simulink model "transmitDSSS_singleUser_USRP"  (R2017a)
settings: Solver=VariableStepAuto  StartTime=0.0  StopTime=inf  RelTol=1e-3
InitFcn:
  | Tb = 1/1000;
  | Tc = 1/8000;
  | fs = 64e3;
  | Ts = 1/fs;
libraries: commfilt2 x2, dspsrcs4 x2, commdigbbndpm3 x1, commsdrhw_v2 x1
settings Model: Creator=prust  LastModifiedBy=prust

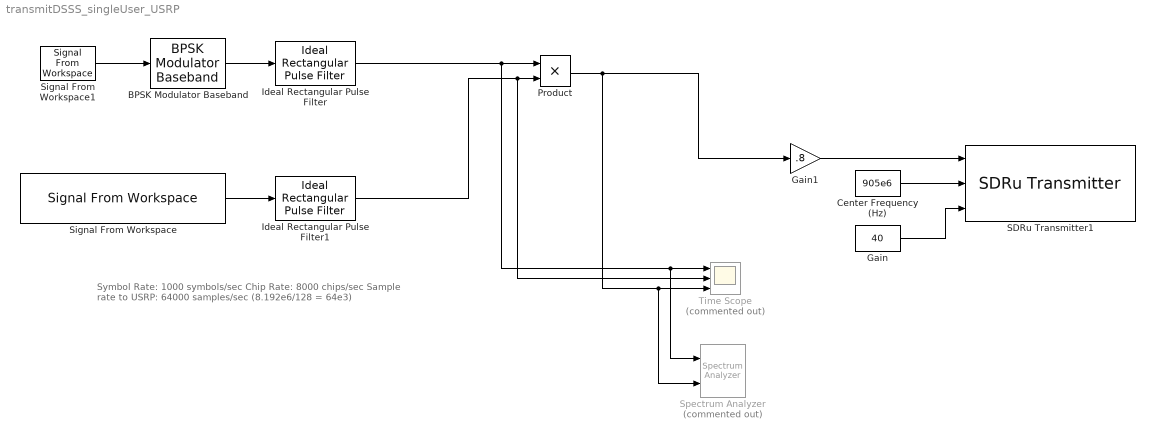
== system transmitDSSS_singleUser_USRP ==
  note: Symbol Rate: 1000 symbols/sec
      | Chip Rate: 8000 chips/sec
      |
      | Sample rate to USRP: 64000 samples/sec
      | (8.192e6/128 = 64e3)
  BPSK Modulator Baseband : commdigbbndpm3/BPSK Modulator Baseband  Ph=0  outDtype=double  outWordLen=16  outUDDataType=sfix(16)  outFracLenMode=Best precision  outFracLen=15  outDataTypeStr=double  outLastDataTypeStr=double
  Center Frequency (Hz) : Constant  Value=905e6
  Gain : Constant  Value=40
  Gain1 : Gain  Gain=.8
  Ideal Rectangular Pulse Filter : commfilt2/Ideal Rectangular Pulse Filter  pulseLen=Tb/Ts  pulseDelay=0  InputProcessing=Columns as channels (frame based)  RateOptions=Allow multirate processing  sampMode=Mute  normCheck=off  normMode=Sum of samples  filterGain=1  saveAsFlag=0  roundingMode=Floor  overflowMode=off  firstCoeffDataTypeStr=Inherit: Same word length as input  firstCoeffMin=[]  firstCoeffMax=[]  firstCoeffLastDataTypeStr=Inherit: Same word length as input  outputDataTypeStr=Inherit: Same as accumulator  outputMin=[]  outputMax=[]  outputLastDataTypeStr=Inherit: Same as accumulator
      settings: SourceProductName=Communications System Toolbox  SourceProductBaseCode=CM
  Ideal Rectangular Pulse Filter1 : commfilt2/Ideal Rectangular Pulse Filter  pulseLen=Tc/Ts  pulseDelay=0  InputProcessing=Columns as channels (frame based)  RateOptions=Allow multirate processing  sampMode=Mute  normCheck=off  normMode=Sum of samples  filterGain=1  saveAsFlag=0  roundingMode=Floor  overflowMode=off  firstCoeffDataTypeStr=Inherit: Same word length as input  firstCoeffMin=[]  firstCoeffMax=[]  firstCoeffLastDataTypeStr=Inherit: Same word length as input  outputDataTypeStr=Inherit: Same as accumulator  outputMin=[]  outputMax=[]  outputLastDataTypeStr=Inherit: Same as accumulator
      settings: SourceProductName=Communications System Toolbox  SourceProductBaseCode=CM
  Product : Product
  SDRu Transmitter1 : commsdrhw_v2/SDRu Transmitter  SourceLibraryInfo="This block requires <a href=\"http://www.mathworks.com/hardware-support/usrp.html\">Communications System Toolbox Support Package for USRP Radio</a>"  rxtx=tx  platform=B200  USRP2_IP='192.168.10.2'  USRP_IP_X300='192.168.10.2'  USRP_IP_X310='192.168.10.2'  USRP_serialNumB200='30703A1'  USRP_serialNumB210=''  ChannelMapping=1  centerFrequency=904e6  centerFrequencySrc=Input port  loOffset=0  loOffsetSrc=Dialog  PPSSource=Internal  clockSource=Internal  masterClkRateB200=8.192e6  masterClkRateB210=32e6  masterClkRateX300=200e6  masterClkRateX310=200e6  masterClkRateParam=8192000  gain=60  gainSrc=Input port  decimInterp=128  decimInterpSrc=Dialog  TransportDataType=int16  USRP2_IP_NUM=[51 48 55 48 51 65 49]  frameLength=362  outputDatatype=Same as transport data type  overrunUnderrunPort=off  sampleTime=1  dboardInfo=|  HOST_DATA_PORT=30000  HOST_CONTROL_PORT=30001  USRP2_DATA_PORT=32769  USRP2_CONTROL_PORT=32768  bufferMode=Continuous streaming  EnableBurstMode=off  NumFramesInBurst=100  USRP_ID='30703A1'
      | dbid: 0
      |           dbName: 'no db found'
      |          freqMin: 0
      |          freqMax: 0
      |          gainMin: 0
      |          gainMax: 0
      |     gainStepSize: 0
      settings: SourceProductName=Communications System Toolbox Support Package for USRP(R) Radio  SourceProductBaseCode=USRP
  Signal From Workspace : dspsrcs4/Signal From Workspace  X=[-1 1 -1 1 1 1 -1 1 1 -1 -1 -1 1 1 1 1]  Ts=Tc  nsamps=1600  OutputAfterFinalValue=Cyclic repetition  ignoreOrWarnInputAndFrameLengths=off  OutputFrames=off
  Signal From Workspace1 : dspsrcs4/Signal From Workspace  X=message  Ts=Tb  nsamps=1600  OutputAfterFinalValue=Cyclic repetition  ignoreOrWarnInputAndFrameLengths=off  OutputFrames=off
  Spectrum Analyzer : SpectrumAnalyzer  Commented=on  NumInputPorts=2
  Time Scope : Scope  Commented=on  NumInputPorts=3
  wires:
  Signal From Workspace1/1 -> BPSK Modulator Baseband/1
  BPSK Modulator Baseband/1 -> Ideal Rectangular Pulse Filter/1
  Ideal Rectangular Pulse Filter/1 -> Spectrum Analyzer/1, Time Scope/1, Product/1
  Gain/1 -> SDRu Transmitter1/3
  Center Frequency (Hz)/1 -> SDRu Transmitter1/2
  Gain1/1 -> SDRu Transmitter1/1
  Ideal Rectangular Pulse Filter1/1 -> Time Scope/2, Product/2
  Product/1 -> Spectrum Analyzer/2, Time Scope/3, Gain1/1
  Signal From Workspace/1 -> Ideal Rectangular Pulse Filter1/1
